simulink model "lab1_1"  (R2023b)
settings: Solver=FixedStepAuto  StartTime=0.0  StopTime=10.0  FixedStep=0.001  RelTol=1e-3
undefined symbols (not defined in the file): a_0, a_1, a_2, b_0, b_1, b_2
settings Model: Creator=nsukh  LastModifiedBy=nsukh

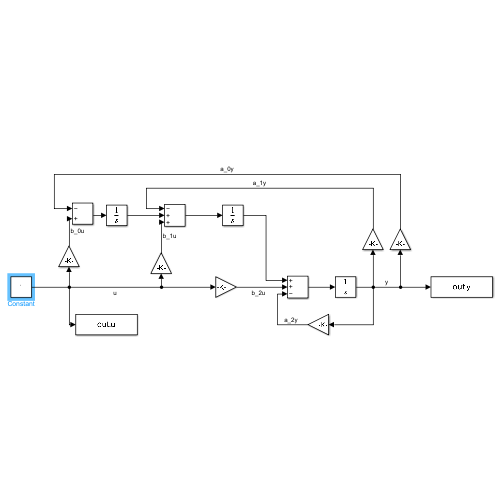
[thumbnail: Simulink's stored preview of the top-level diagram]
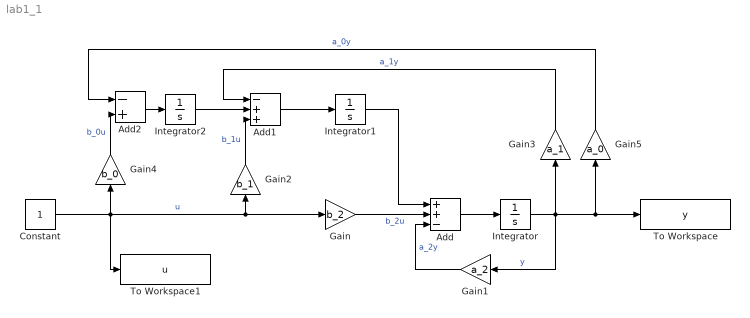
== system lab1_1 ==
  Add : Sum  Inputs=++-
  Add1 : Sum  Inputs=-++
  Add2 : Sum  Inputs=-+
  Constant : Constant  SampleTime=-1
  Gain : Gain  Gain=b_2
  Gain1 : Gain  Gain=a_2
  Gain2 : Gain  Gain=b_1
  Gain3 : Gain  Gain=a_1
  Gain4 : Gain  Gain=b_0
  Gain5 : Gain  Gain=a_0
  Integrator : Integrator
  Integrator1 : Integrator
  Integrator2 : Integrator
  To Workspace : ToWorkspace  VariableName=y  SaveFormat=Timeseries  SampleTime=-1
  To Workspace1 : ToWorkspace  VariableName=u  SaveFormat=Timeseries  SampleTime=-1
  wires:
  Integrator/1 -> To Workspace/1, Gain5/1, Gain1/1, Gain3/1  "y"
  Constant/1 -> To Workspace1/1, Gain2/1, Gain/1, Gain4/1  "u"
  Gain/1 -> Add/2  "b_2u"
  Add/1 -> Integrator/1
  Gain1/1 -> Add/3  "a_2y"
  Integrator1/1 -> Add/1
  Add1/1 -> Integrator1/1
  Gain2/1 -> Add1/3  "b_1u"
  Gain3/1 -> Add1/1  "a_1y"
  Integrator2/1 -> Add1/2
  Gain4/1 -> Add2/2  "b_0u"
  Add2/1 -> Integrator2/1
  Gain5/1 -> Add2/1  "a_0y"
